simulink model "Prova_skew_simmetric"  (R2015a)
settings: Solver=ode45  StartTime=0.0  StopTime=10.0  RelTol=1e-3
undefined symbols (not defined in the file or in its folder): I_Pi, Kq, omega_hover
libraries: aerolibutil x1
settings Model: Creator=Claudio  LastModifiedBy=Claudio

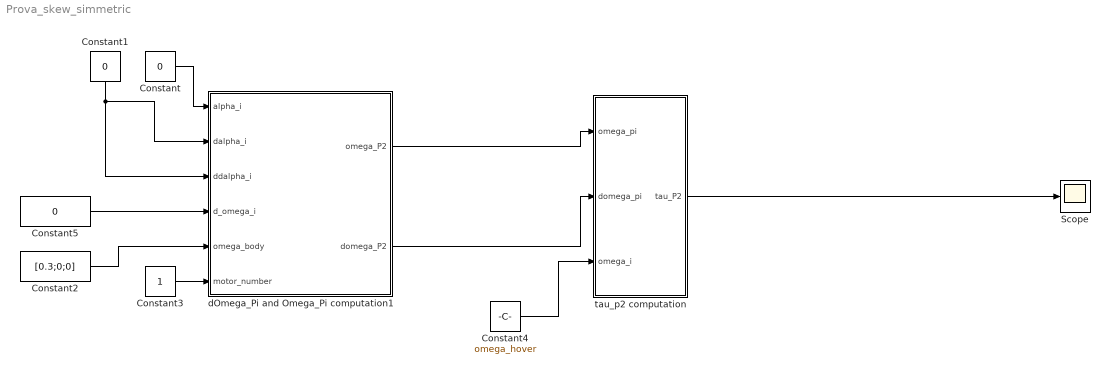
== system Prova_skew_simmetric ==
  Constant : Constant  Value=0
  Constant1 : Constant  Value=0
  Constant2 : Constant  Value=[0.3;0;0]
  Constant3 : Constant
  Constant4 : Constant  Value=omega_hover
  Constant5 : Constant  Value=0
  Scope : Scope
  dOmega_Pi and Omega_Pi computation1 : Subsystem
  tau_p2 computation : Subsystem
  wires:
  Constant/1 -> dOmega_Pi and Omega_Pi computation1/1(alpha_i)
  Constant1/1 -> dOmega_Pi and Omega_Pi computation1/3(ddalpha_i), dOmega_Pi and Omega_Pi computation1/2(dalpha_i)
  Constant2/1 -> dOmega_Pi and Omega_Pi computation1/5(omega_body)
  dOmega_Pi and Omega_Pi computation1/1(omega_P2) -> tau_p2 computation/1(omega_pi)
  dOmega_Pi and Omega_Pi computation1/2(domega_P2) -> tau_p2 computation/2(domega_pi)
  tau_p2 computation/1(tau_P2) -> Scope/1
  Constant3/1 -> dOmega_Pi and Omega_Pi computation1/6(motor_number)
  Constant4/1 -> tau_p2 computation/3(omega_i)
  Constant5/1 -> dOmega_Pi and Omega_Pi computation1/4(d_omega_i)

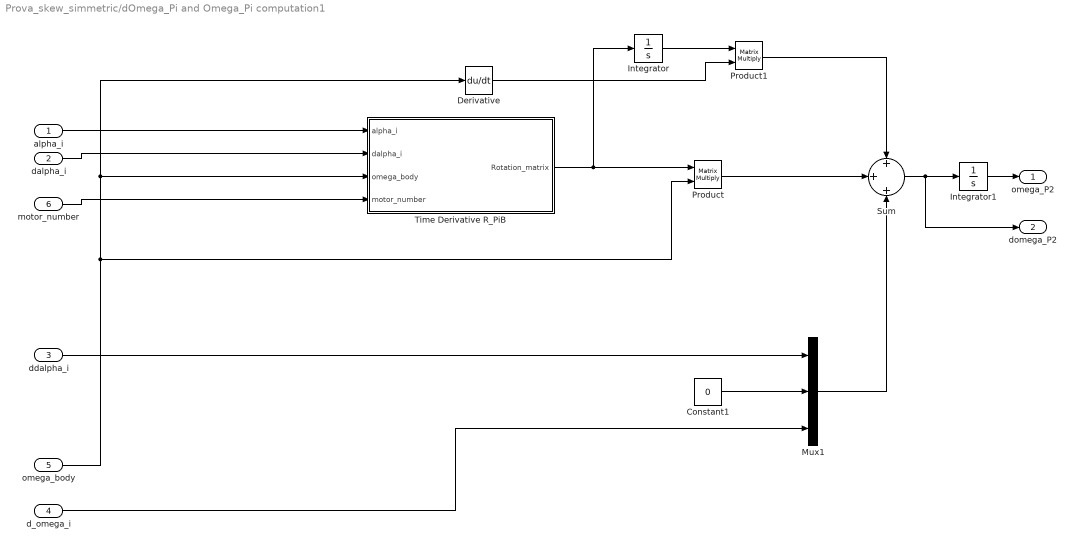
== system Prova_skew_simmetric/dOmega_Pi and Omega_Pi computation1 ==
  alpha_i : Inport
  dalpha_i : Inport  Port=2
  ddalpha_i : Inport  Port=3
  d_omega_i : Inport  Port=4
  omega_body : Inport  Port=5
  motor_number : Inport  Port=6
  Constant1 : Constant  Value=0
  Derivative : Derivative
  Integrator : Integrator
  Integrator1 : Integrator
  Mux1 : Mux  Inputs=3
  Product : Product  Multiplication=Matrix(*)
  Product1 : Product  Multiplication=Matrix(*)
  Sum : Sum  Inputs=+|+|+
  Time Derivative R_PiB : MATLAB Function  TreatAsAtomicUnit=on
  omega_P2 : Outport
  domega_P2 : Outport  Port=2
  wires:
  Derivative/1 -> Product1/2
  Product/1 -> Sum/2
  Time Derivative R_PiB/1(Rotation_matrix) -> Integrator/1, Product/1
  Constant1/1 -> Mux1/2
  omega_body/1 -> Product/2, Time Derivative R_PiB/3(omega_body), Derivative/1
  dalpha_i/1 -> Time Derivative R_PiB/2(dalpha_i)
  alpha_i/1 -> Time Derivative R_PiB/1(alpha_i)
  Integrator/1 -> Product1/1
  d_omega_i/1 -> Mux1/3
  Sum/1 -> domega_P2/1, Integrator1/1
  Product1/1 -> Sum/1
  Mux1/1 -> Sum/3
  Integrator1/1 -> omega_P2/1
  ddalpha_i/1 -> Mux1/1
  motor_number/1 -> Time Derivative R_PiB/4(motor_number)

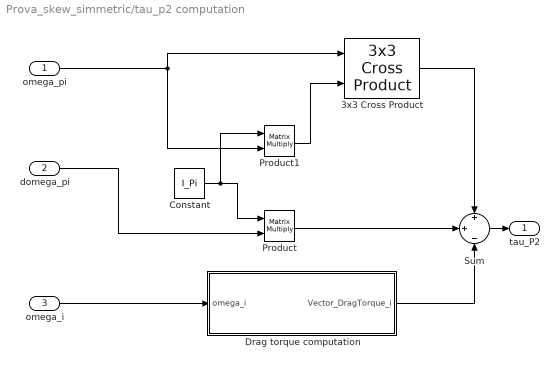
== system Prova_skew_simmetric/tau_p2 computation ==
  omega_pi : Inport
  domega_pi : Inport  Port=2
  omega_i : Inport  Port=3
  3x3 Cross Product : aerolibutil/3x3 Cross Product
  Constant : Constant  Value=I_Pi
  Drag torque computation : Subsystem
  Product : Product  Multiplication=Matrix(*)
  Product1 : Product  Multiplication=Matrix(*)
  Sum : Sum  Inputs=+|+|-
  tau_P2 : Outport
  wires:
  3x3 Cross Product/1 -> Sum/1
  Sum/1 -> tau_P2/1
  Product1/1 -> 3x3 Cross Product/2
  domega_pi/1 -> Product/2
  Product/1 -> Sum/2
  omega_pi/1 -> Product1/2, 3x3 Cross Product/1
  Constant/1 -> Product/1, Product1/1
  omega_i/1 -> Drag torque computation/1(omega_i)
  Drag torque computation/1(Vector_DragTorque_i) -> Sum/3

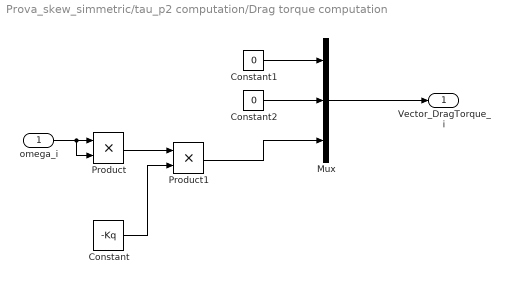
== system Prova_skew_simmetric/tau_p2 computation/Drag torque computation ==
  omega_i : Inport
  Constant : Constant  Value=-Kq
  Constant1 : Constant  Value=0
  Constant2 : Constant  Value=0
  Mux : Mux  Inputs=3
  Product : Product
  Product1 : Product
  Vector_DragTorque_i : Outport
  wires:
  Constant2/1 -> Mux/2
  omega_i/1 -> Product/2, Product/1
  Product/1 -> Product1/1
  Constant1/1 -> Mux/1
  Mux/1 -> Vector_DragTorque_i/1
  Product1/1 -> Mux/3
  Constant/1 -> Product1/2

== matlab function Prova_skew_simmetric/dOmega_Pi and Omega_Pi computation1/Time Derivative R_PiB ==
  data: alpha_i input; dalpha_i input; omega_body input; Rotation_matrix output; motor_number input
function Rotation_matrix = fcn(alpha_i,dalpha_i,omega_body,motor_number)
%#codegen

% Rotation matrix from Body to propeller group
psi = (motor_number-1)*pi/2;
phi = alpha_i;
dphi = dalpha_i;
% R_PiB = [cos(psi),           sin(psi),        0;
%        -cos(phi)*sin(psi),  cos(phi)*cos(psi), sin(phi);
%         sin(phi)*sin(psi), -cos(psi)*sin(phi), cos(phi)];
% dR_PiB = [ 0, 0, 0 ;
%     sin(phi)*sin(psi)*dphi, -sin(phi)*cos(psi)*dphi, cos(phi)*dphi;
%     cos(phi)*sin(psi)*dphi, -cos(phi)*sin(psi)*dphi, -sin(phi)*dphi ];
omega_x = omega_body(1);
omega_y = omega_body(2);
omega_z = omega_body(3);

% Define the skew simmetric matrix
S = [0 -omega_z omega_y;omega_z 0 -omega_x; -omega_y omega_x 0];

R_PiB = [cos(psi),           sin(psi),        0;
       -cos(phi)*sin(psi),  cos(phi)*cos(psi), sin(phi);
        sin(phi)*sin(psi), -cos(psi)*sin(phi), cos(phi)];

dR_PiB = S*R_PiB;


Rotation_matrix = dR_PiB
